simulink model "ParameterIdentification"  (R2024b)
settings: Solver=FixedStepAuto  StartTime=0.0  StopTime=3  FixedStep=1e-6  MaxStep=1e-6  RelTol=1e-3
undefined symbols (not defined in the file): F1, Period, Pn, Ts, U_ref, Udc
libraries: My_library x3, spsDCVoltageSourceLib x1, spsGroundLib x1, simulink x1, spsPermanentMagnetSynchronousMachineLib x1, spsTwoLevelConverterLib x1, sps_lib x1
(part 1 of 2)
settings Model: DataDictionary=Based_FOC_Data.sldd  Creator=sa127  LastModifiedBy=sa127
settings OptimizationCC: DefaultParameterBehavior=Inlined  UseDivisionForNetSlopeComputation=on  GainParamInheritBuiltInType=on  UseFloatMulNetSlope=on  InlineInvariantSignals=on  PassReuseOutputArgsAs=Individual arguments  ZeroExternalMemoryAtStartup=off  ZeroInternalMemoryAtStartup=off  NoFixptDivByZeroProtection=on  EfficientFloat2IntCast=on  LifeSpan=1  OptimizeBlockOrder=speed  DifferentSizesBufferReuse=on  MultiThreadedLoops=on  EfficientTunableParamExpr=on
settings DebuggingCC: ParamSuppressDoubleToSinglePrecisionLossMsg=on  ParameterTunabilityLossMsg=error
settings HardwareCC: ProdBitPerPointer=32  ProdBitPerSizeT=32  ProdBitPerPtrDiffT=32  ProdLargestAtomicInteger=Long  ProdLargestAtomicFloat=Double  ProdWordSize=32  ProdLongLongMode=on  ProdHWDeviceType=ARM Compatible->ARM Cortex-M
settings SFSimCC: MATLABDynamicMemAlloc=off
settings RTWCC: Description=Embedded Coder  SystemTargetFile=ert.tlc  TemplateMakefile=ert_default_tmf  GenerateReport=on  IncludeHyperlinkInReport=on  LaunchReport=on  GenerateTraceInfo=on  GenerateTraceReport=on  GenerateTraceReportSl=on  GenerateTraceReportSf=on  GenerateTraceReportEml=on  GenerateWebview=on  GenerateCodeMetricsReport=on  GenerateCodeReplacementReport=on
settings CodeAppCC: ForceParamTrailComments=on  IgnoreCustomStorageClasses=off  OperatorAnnotations=on  SimulinkDataObjDesc=on  SFDataObjDesc=on  CustomSymbolStrGlobalVar=rt$N$M  CustomSymbolStrType=$N$M  CustomSymbolStrFcn=$N$M$F  CustomSymbolStrMacro=$N$M  InsertBlockDesc=on
settings ERTTargetCC: TargetLangStandard=C99 (ISO)  CodeReplacementLibrary=ARM Cortex-M  GenerateSampleERTMain=on  IncludeMdlTerminateFcn=off  CombineSignalStateStructs=on  SupportComplex=off  SupportNonInlinedSFcns=on  ERTCustomFileTemplate=example_file_process.tlc  ERTFilePackagingFormat=CompactWithDataFile

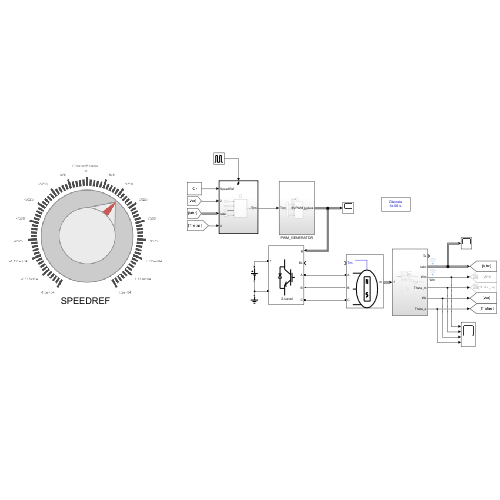
[thumbnail: Simulink's stored preview of the top-level diagram]
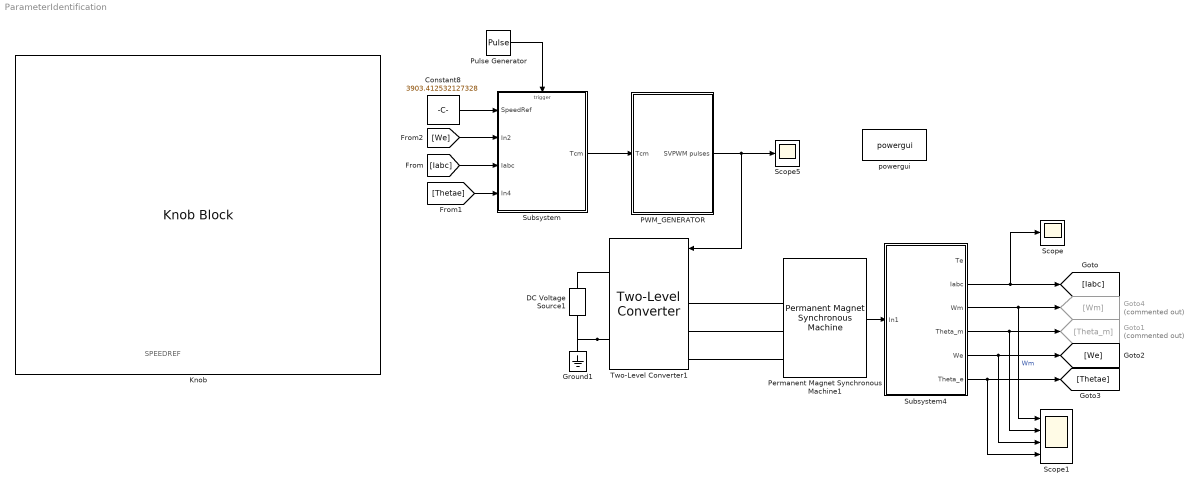
== system ParameterIdentification ==
  note: SPEEDREF
  Constant8 : Constant  Value=3903.412532127328
  DC Voltage Source1 : spsDCVoltageSourceLib/DC Voltage Source  Amplitude=300  Measurements=None
  Goto1 : Goto  Commented=on  GotoTag=Theta_m
  Goto4 : Goto  Commented=on  GotoTag=Wm
  Ground1 : spsGroundLib/Ground  LConnTagsString=a
  Knob : KnobBlock  ScaleMin=-15000  ScaleMax=15000
  PWM_GENERATOR : Subsystem
  Permanent Magnet Synchronous Machine1 : spsPermanentMagnetSynchronousMachineLib/Permanent Magnet Synchronous Machine  NbPhases=3  FluxDistribution=Sinusoidal  RotorType=Salient-pole  MechanicalLoad=Torque Tm  PresetModel="04:  6 Nm 300 Vdc 4500 RPM - 6 Nm"  ShowDetailedParameters=on  MeasurementBus=on  Resistance=0.62  Inductance=8.5e-3  dqInductances=[0.001971 0.002179]  La=0.002075  MachineConstant=Flux linkage established by magnets (V.s)  Flux=0.08627  VoltageCst=67.038  TorqueCst=0.5544  Flat=120  Mechanical=[0.0003617 9.444e-05 4 0]  PolePairs=4  InitialConditions=[0,0, 0,0]  InitialConditions5ph=[0 0 0 0 0 0]  RefAngle=Aligned with phase A axis (original Park)  IterativeDiscreteModel=Trapezoidal non iterative  TsBlock=-1  TsPowergui=0
  Pulse Generator : DiscretePulseGenerator  PulseType=Time based  Period=0.0001  PulseWidth=50
  Scope : Scope
  Scope1 : Scope  NumInputPorts=4
  Scope5 : Scope
  Subsystem : Subsystem
  Subsystem4 : Subsystem
  Two-Level Converter1 : spsTwoLevelConverterLib/Two-Level Converter  ModelType=Switching function  Ron=1e-3  Rs=1e6  Cs=inf  Vforward=[0,0]  Ron_Diode=1e-3  Rs_Diode=1e6  Cs_Diode=inf  Vf_Diode=1e-3  Rs_CurrentSource=inf  Ron_ACsource=1e-3
      settings: LibrarySourceBlock=sps_lib/Power Electronics/Two-Level Converter
  powergui : sps_lib/powergui  Priority=1  SimulationMode=Discrete  SampleTime=0.000001  frequency=60  Iterations=50  frequencyindice=0  Pbase=100e6  ErrMax=1e-4  UnitsV=kV  UnitsW=MW  buscounter=0  FunctionMessages=off  echomessages=off  EnableUseOfTLC=off  CurrentSourceSwitches=off  DisableSnubberDevices=off  DisableRonSwitches=off  DisableVfSwitches=off  DisplayEquations=off  AutomaticDiscreteSolvers=off  SolverType=Tustin/Backward Euler (TBE)  Interpol=off  ExternalGateDelay=off  methode=off  Ts=100  x0status=blocks  SPID=on  SwTol=0  HookPort=off  NonlinearTolerance=1e-4  nMaxIteration=100  ContinueOnMaxIteration=off  RestoreLinks=warning  ResistiveCurrentMeasurement=off  Frange=[0:2:500]  Ylog=off  Xlog=on  ShowGrid=off  save=off  variable=ZData  structure=0  ZoomFFT=off  StartTime=0.0  cycles=1  DisplayStyle=1  fundamental=60  FreqAxis=off  MaxFrequency=1000  frequencyindicesteady=1  RmsSteady=1  display=off
  wires:
  Permanent Magnet Synchronous Machine1/1 -> Subsystem4/1(In1)
  Subsystem4/2(Iabc) -> Scope/1, [Iabc]
  Subsystem4/3(Wm) -> Scope1/1, Goto4/1  "Wm"
  Subsystem4/4(Theta_m) -> Goto1/1, Scope1/2
  Subsystem4/5(We) -> Scope1/3, [We]
  Subsystem4/6(Theta_e) -> Scope1/4, [Thetae]
  PWM_GENERATOR/1(SVPWM pulses) -> Scope5/1, Two-Level Converter1/1
  Constant8/1 -> Subsystem/1(SpeedRef)
  [We] -> Subsystem/2(In2)
  [Iabc] -> Subsystem/3(Iabc)
  [Thetae] -> Subsystem/4(In4)
  Pulse Generator/1 -> Subsystem/Trigger
  Subsystem/1(Tcm) -> PWM_GENERATOR/1(Tcm)
  connections:
  Two-Level Converter1/RConn2 -- DC Voltage Source1/LConn1 -- Ground1/LConn1
  Two-Level Converter1/LConn2 -- Permanent Magnet Synchronous Machine1/LConn2
  Two-Level Converter1/LConn1 -- Permanent Magnet Synchronous Machine1/LConn1
  Two-Level Converter1/LConn3 -- Permanent Magnet Synchronous Machine1/LConn3
  DC Voltage Source1/RConn1 -- Two-Level Converter1/RConn1

== system ParameterIdentification/PWM_GENERATOR ==
  Tcm : Inport
  Demux : Demux  Outputs=3
  Scope1 : Scope  NumInputPorts=3
  Subsystem1 : Subsystem
  SVPWM pulses : Outport
  wires:
  Demux/1 -> Subsystem1/1(Tcm1), Scope1/1
  Demux/2 -> Subsystem1/2(Tcm2), Scope1/2
  Demux/3 -> Subsystem1/3(Tcm3), Scope1/3
  Subsystem1/1(SVPWM pulses) -> SVPWM pulses/1
  Tcm/1 -> Demux/1

== system ParameterIdentification/Subsystem ==
  SpeedRef : Inport
  In2 : Inport  Port=2
  Iabc : Inport  Port=3
  In4 : Inport  Port=4
  Trigger : TriggerPort  VariantControl=(inherit)  PortDimensions=1
  Sensorless : Subsystem
  Tcm : Outport
  wires:
  SpeedRef/1 -> Sensorless/1(SpeedRef)
  In2/1 -> Sensorless/2(In2)
  In4/1 -> Sensorless/4(In4)
  Iabc/1 -> Sensorless/3(Iabc)
  Sensorless/1(Tcm) -> Tcm/1

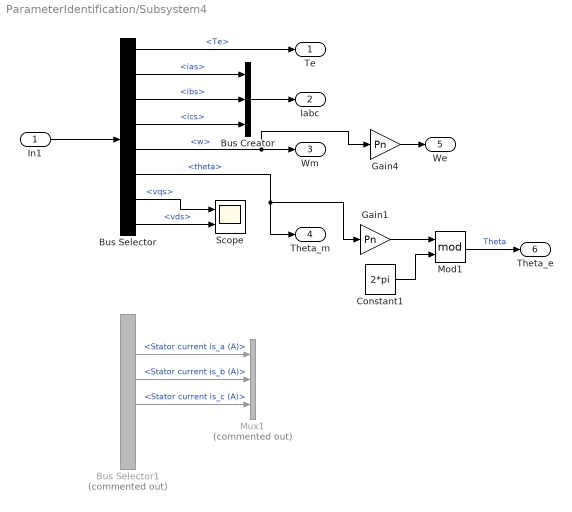
== system ParameterIdentification/Subsystem4 ==
  In1 : Inport
  Bus Creator : BusCreator  Inputs=3
  Bus Selector : BusSelector  OutputSignals=Te,ias,ibs,ics,w,theta,vqs,vds
  Bus Selector1 : BusSelector  Commented=on  OutputSignals=Electromagnetic torque Te (N*m),Stator current is_a (A),Stator current is_b (A),Stator current is_c (A),Rotor speed wm (rad/s),Rotor angle thetam (rad)
  Constant1 : Constant  Value=2*pi
  Gain1 : Gain  Gain=Pn
  Gain4 : Gain  Gain=Pn
  Mod1 : Math  Operator=mod
  Mux1 : Mux  Commented=on  Inputs=3
  Scope : Scope  NumInputPorts=2
  Te : Outport
  Iabc : Outport  Port=2
  Wm : Outport  Port=3
  Theta_m : Outport  Port=4
  We : Outport  Port=5
  Theta_e : Outport  Port=6
  wires:
  Bus Selector/2 -> Bus Creator/1  "<ias>"
  Bus Selector/4 -> Bus Creator/3  "<ics>"
  Bus Selector/3 -> Bus Creator/2  "<ibs>"
  Bus Selector1/4 -> Mux1/3  "<Stator current is_c (A)>"
  Bus Selector1/3 -> Mux1/2  "<Stator current is_b (A)>"
  Bus Selector1/2 -> Mux1/1  "<Stator current is_a (A)>"
  In1/1 -> Bus Selector/1
  Bus Selector/1 -> Te/1  "<Te>"
  Bus Selector/5 -> Gain4/1, Wm/1  "<w>"
  Bus Selector/6 -> Gain1/1, Theta_m/1  "<theta>"
  Bus Selector/8 -> Scope/2  "<vds>"
  Bus Selector/7 -> Scope/1  "<vqs>"
  Constant1/1 -> Mod1/2
  Gain1/1 -> Mod1/1
  Gain4/1 -> We/1
  Mod1/1 -> Theta_e/1  "Theta"
  Bus Creator/1 -> Iabc/1

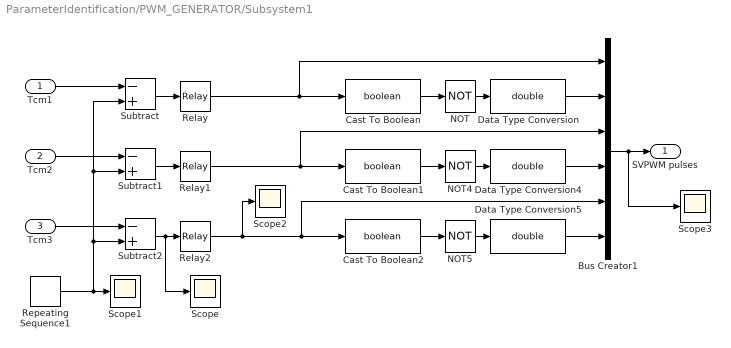
== system ParameterIdentification/PWM_GENERATOR/Subsystem1 ==
  Tcm1 : Inport
  Tcm2 : Inport  Port=2
  Tcm3 : Inport  Port=3
  Bus Creator1 : BusCreator  Inputs=6
  Cast To Boolean : DataTypeConversion  OutDataTypeStr=boolean  SaturateOnIntegerOverflow=off  RndMeth=Floor
  Cast To Boolean1 : DataTypeConversion  OutDataTypeStr=boolean  SaturateOnIntegerOverflow=off  RndMeth=Floor
  Cast To Boolean2 : DataTypeConversion  OutDataTypeStr=boolean  SaturateOnIntegerOverflow=off  RndMeth=Floor
  Data Type Conversion : DataTypeConversion  OutDataTypeStr=double  SaturateOnIntegerOverflow=off  RndMeth=Floor
  Data Type Conversion4 : DataTypeConversion  OutDataTypeStr=double  SaturateOnIntegerOverflow=off  RndMeth=Floor
  Data Type Conversion5 : DataTypeConversion  OutDataTypeStr=double  SaturateOnIntegerOverflow=off  RndMeth=Floor
  NOT : Logic  Operator=NOT  IconShape=distinctive  AllPortsSameDT=off  OutDataTypeStr=boolean
  NOT4 : Logic  Operator=NOT  IconShape=distinctive  AllPortsSameDT=off  OutDataTypeStr=boolean
  NOT5 : Logic  Operator=NOT  IconShape=distinctive  AllPortsSameDT=off  OutDataTypeStr=boolean
  Relay : Relay
  Relay1 : Relay
  Relay2 : Relay
  Repeating Sequence1 : simulink/Sources/Repeating Sequence  rep_seq_t=[0 Ts/2 Ts]  rep_seq_y=[0 Period/2 0]
  Scope{,1..3} (4 alike) : Scope
  Subtract : Sum  Inputs=-+
  Subtract1 : Sum  Inputs=-+
  Subtract2 : Sum  Inputs=-+
  SVPWM pulses : Outport
  wires:
  Tcm3/1 -> Subtract2/1
  Cast To Boolean/1 -> NOT/1
  Subtract/1 -> Relay/1
  Relay2/1 -> Scope2/1, Bus Creator1/5, Cast To Boolean2/1
  Subtract2/1 -> Scope/1, Relay2/1
  Cast To Boolean2/1 -> NOT5/1
  Subtract1/1 -> Relay1/1
  Repeating Sequence1/1 -> Subtract2/2, Subtract1/2, Subtract/2, Scope1/1
  Tcm1/1 -> Subtract/1
  NOT/1 -> Data Type Conversion/1
  Cast To Boolean1/1 -> NOT4/1
  Bus Creator1/1 -> Scope3/1, SVPWM pulses/1
  NOT5/1 -> Data Type Conversion5/1
  Relay1/1 -> Bus Creator1/3, Cast To Boolean1/1
  Relay/1 -> Bus Creator1/1, Cast To Boolean/1
  Tcm2/1 -> Subtract1/1
  Data Type Conversion5/1 -> Bus Creator1/6
  Data Type Conversion/1 -> Bus Creator1/2
  NOT4/1 -> Data Type Conversion4/1
  Data Type Conversion4/1 -> Bus Creator1/4

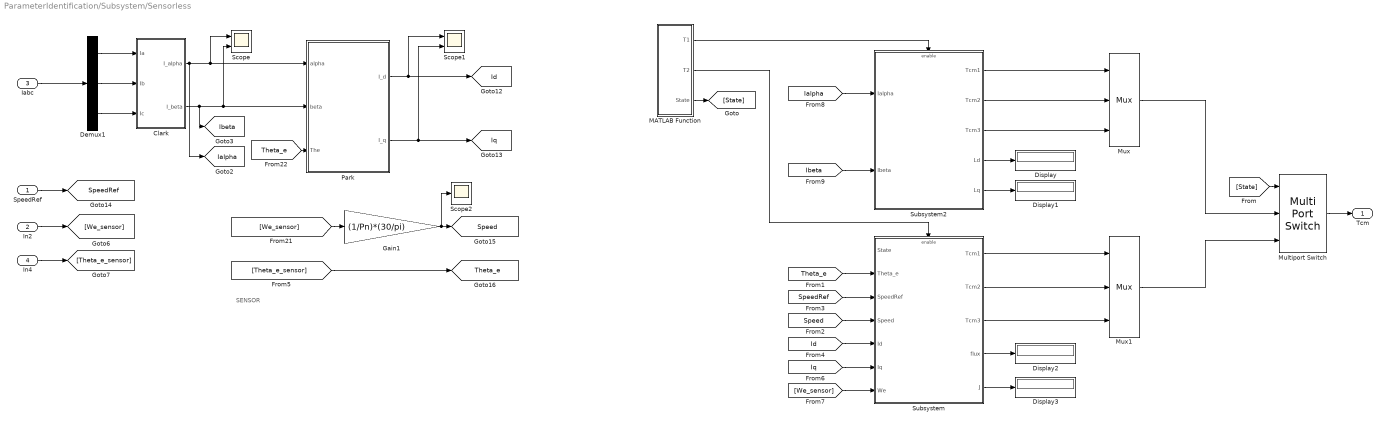
== system ParameterIdentification/Subsystem/Sensorless ==
  note: SENSOR
  SpeedRef : Inport
  In2 : Inport  Port=2
  Iabc : Inport  Port=3
  In4 : Inport  Port=4
  Clark : Subsystem
  Demux1 : Demux  Outputs=3
  Display{,1..3} (4 alike) : Display
  Gain1 : Gain  Gain=(1/Pn)*(30/pi)
  MATLAB Function : MATLAB Function  TreatAsAtomicUnit=on
  Multiport Switch : MultiPortSwitch  Inputs=2  SaturateOnIntegerOverflow=off  InputSameDT=off
  Mux : Mux  Inputs=3
  Mux1 : Mux  Inputs=3
  Park : Subsystem
  Scope : Scope  NumInputPorts=2
  Scope1 : Scope  NumInputPorts=2
  Scope2 : Scope
  Subsystem : Subsystem
  Subsystem2 : Subsystem
  Tcm : Outport
  tag scope: Ialpha=global, Ibeta=global, Id=global, Iq=global, Speed=global, SpeedRef=global, Theta_e=global
  wires:
  Park/1(I_d) -> [Id], Scope1/1
  Demux1/3 -> Clark/3(Ic)
  Demux1/1 -> Clark/1(Ia)
  Iabc/1 -> Demux1/1
  Clark/1(I_alpha) -> [Ialpha], Scope/1, Park/1(alpha)
  Clark/2(I_beta) -> [Ibeta], Scope/2, Park/2(beta)
  Park/2(I_q) -> [Iq], Scope1/2
  Demux1/2 -> Clark/2(Ib)
  [We_sensor] -> Gain1/1
  In2/1 -> [We_sensor]
  In4/1 -> [Theta_e_sensor]
  SpeedRef/1 -> [SpeedRef]
  Gain1/1 -> Scope2/1, [Speed]
  [Theta_e_sensor] -> [Theta_e]
  [Theta_e] -> Park/3(The)
  Mux/1 -> Multiport Switch/2
  Mux1/1 -> Multiport Switch/3
  Subsystem/1(Tcm1) -> Mux1/1
  Subsystem/2(Tcm2) -> Mux1/2
  Subsystem/3(Tcm3) -> Mux1/3
  MATLAB Function/2(T2) -> Subsystem/Enable
  MATLAB Function/3(State) -> [State]
  [State] -> Multiport Switch/1
  [Theta_e] -> Subsystem/2(Theta_e)
  [SpeedRef] -> Subsystem/3(SpeedRef)
  [Speed] -> Subsystem/4(Speed)
  [Id] -> Subsystem/5(Id)
  [Iq] -> Subsystem/6(Iq)
  [We_sensor] -> Subsystem/7(We)
  Multiport Switch/1 -> Tcm/1
  [Ialpha] -> Subsystem2/1(Ialpha)
  [Ibeta] -> Subsystem2/2(Ibeta)
  Subsystem2/1(Tcm1) -> Mux/1
  Subsystem2/2(Tcm2) -> Mux/2
  Subsystem2/3(Tcm3) -> Mux/3
  MATLAB Function/1(T1) -> Subsystem2/Enable
  Subsystem2/4(Ld) -> Display/1
  Subsystem2/5(Lq) -> Display1/1
  Subsystem/4(flux) -> Display2/1
  Subsystem/5(J) -> Display3/1

== system ParameterIdentification/Subsystem/Sensorless/Clark ==
  Ia : Inport
  Ib : Inport  Port=2
  Ic : Inport  Port=3
  Fcn : Fcn  Expr=(u(1)-0.5*u(2)-0.5*u(3))*2/3
  Fcn1 : Fcn  Expr=(sqrt(3)/2*u(2)-sqrt(3)/2*u(3))*2/3
  Mux : Mux  Inputs=3
  I_alpha : Outport
  I_beta : Outport  Port=2
  wires:
  Ib/1 -> Mux/2
  Fcn1/1 -> I_beta/1
  Ic/1 -> Mux/3
  Mux/1 -> Fcn1/1, Fcn/1
  Fcn/1 -> I_alpha/1
  Ia/1 -> Mux/1

== system ParameterIdentification/Subsystem/Sensorless/Park ==
  alpha : Inport
  beta : Inport  Port=2
  The : Inport  Port=3
  Fcn : Fcn  Expr=cos(u(3))*u(1)+sin(u(3))*u(2)
  Fcn1 : Fcn  Expr=-sin(u(3))*u(1)+cos(u(3))*u(2)
  Mux : Mux  Inputs=3
  I_d : Outport
  I_q : Outport  Port=2
  wires:
  Fcn/1 -> I_d/1
  Fcn1/1 -> I_q/1
  The/1 -> Mux/3
  alpha/1 -> Mux/1
  Mux/1 -> Fcn1/1, Fcn/1
  beta/1 -> Mux/2

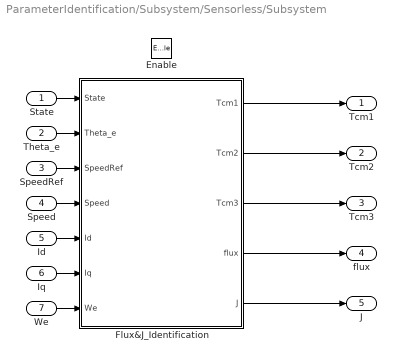
== system ParameterIdentification/Subsystem/Sensorless/Subsystem ==
  State : Inport
  Theta_e : Inport  Port=2
  SpeedRef : Inport  Port=3
  Speed : Inport  Port=4
  Id : Inport  Port=5
  Iq : Inport  Port=6
  We : Inport  Port=7
  Enable : EnablePort
  Flux&J_Identification : Subsystem
  Tcm1 : Outport
  Tcm2 : Outport  Port=2
  Tcm3 : Outport  Port=3
  flux : Outport  Port=4
  J : Outport  Port=5
  wires:
  Flux&J_Identification/1(Tcm1) -> Tcm1/1
  Flux&J_Identification/2(Tcm2) -> Tcm2/1
  State/1 -> Flux&J_Identification/1(State)
  Flux&J_Identification/3(Tcm3) -> Tcm3/1
  Theta_e/1 -> Flux&J_Identification/2(Theta_e)
  We/1 -> Flux&J_Identification/7(We)
  Iq/1 -> Flux&J_Identification/6(Iq)
  Id/1 -> Flux&J_Identification/5(Id)
  Speed/1 -> Flux&J_Identification/4(Speed)
  SpeedRef/1 -> Flux&J_Identification/3(SpeedRef)
  Flux&J_Identification/4(flux) -> flux/1
  Flux&J_Identification/5(J) -> J/1

== system ParameterIdentification/Subsystem/Sensorless/Subsystem2 ==
  Ialpha : Inport
  Ibeta : Inport  Port=2
  Enable : EnablePort
  Subsystem1 : Subsystem
  Tcm1 : Outport
  Tcm2 : Outport  Port=2
  Tcm3 : Outport  Port=3
  Ld : Outport  Port=4
  Lq : Outport  Port=5
  wires:
  Ialpha/1 -> Subsystem1/1(Ialpha)
  Ibeta/1 -> Subsystem1/2(Ibeta)
  Subsystem1/1(Tcm1) -> Tcm1/1
  Subsystem1/3(Tcm3) -> Tcm3/1
  Subsystem1/2(Tcm2) -> Tcm2/1
  Subsystem1/4(Ld) -> Ld/1
  Subsystem1/5(Lq) -> Lq/1

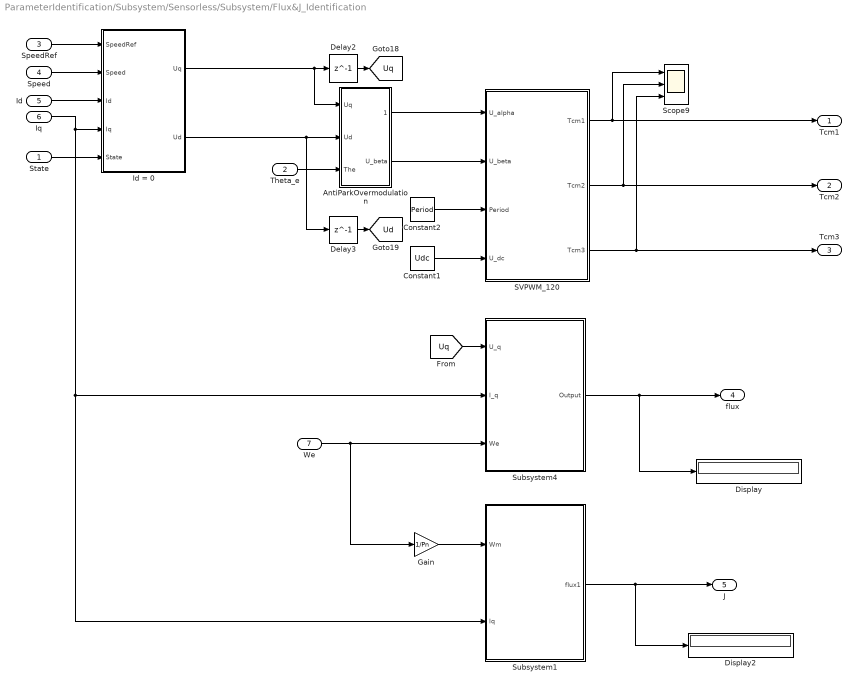
== system ParameterIdentification/Subsystem/Sensorless/Subsystem/Flux&J_Identification ==
  State : Inport
  Theta_e : Inport  Port=2
  SpeedRef : Inport  Port=3
  Speed : Inport  Port=4
  Id : Inport  Port=5
  Iq : Inport  Port=6
  We : Inport  Port=7
  AntiParkOvermodulation : Subsystem
  Constant1 : Constant  Value=Udc
  Constant2 : Constant  Value=Period
  Delay2 : Delay  DelayLength=1
  Delay3 : Delay  DelayLength=1
  Display : Display
  Display2 : Display
  Gain : Gain  Gain=1/Pn
  Id = 0 : Subsystem
  SVPWM_120 : MATLAB Function  TreatAsAtomicUnit=on
  Scope9 : Scope  NumInputPorts=3
  Subsystem1 : Subsystem
  Subsystem4 : Subsystem
  Tcm1 : Outport
  Tcm2 : Outport  Port=2
  Tcm3 : Outport  Port=3
  flux : Outport  Port=4
  J : Outport  Port=5
  tag scope: Ud=global, Uq=global
  wires:
  Iq/1 -> Subsystem4/2(I_q), Subsystem1/2(Iq), Id = 0/4(Iq)
  Id = 0/1(Uq) -> AntiParkOvermodulation/1(Uq), Delay2/1
  Speed/1 -> Id = 0/2(Speed)
  Constant2/1 -> SVPWM_120/3(Period)
  Theta_e/1 -> AntiParkOvermodulation/3(The)
  Gain/1 -> Subsystem1/1(Wm)
  Delay2/1 -> [Uq]
  SVPWM_120/3(Tcm3) -> Tcm3/1, Scope9/3
  Constant1/1 -> SVPWM_120/4(U_dc)
  [Uq] -> Subsystem4/1(U_q)
  SVPWM_120/1(Tcm1) -> Tcm1/1, Scope9/1
  Id/1 -> Id = 0/3(Id)
  SVPWM_120/2(Tcm2) -> Tcm2/1, Scope9/2
  AntiParkOvermodulation/1(U_alpha) -> SVPWM_120/1(U_alpha)
  AntiParkOvermodulation/2(U_beta) -> SVPWM_120/2(U_beta)
  Subsystem1/1(flux1) -> J/1, Display2/1
  We/1 -> Gain/1, Subsystem4/3(We)
  Subsystem4/1(Output) -> flux/1, Display/1
  Delay3/1 -> [Ud]
  Id = 0/2(Ud) -> AntiParkOvermodulation/2(Ud), Delay3/1
  SpeedRef/1 -> Id = 0/1(SpeedRef)
  State/1 -> Id = 0/5(State)

== system ParameterIdentification/Subsystem/Sensorless/Subsystem2/Subsystem1 ==
  Ialpha : Inport
  Ibeta : Inport  Port=2
  Subsystem : Subsystem
  Tcm1 : Outport
  Tcm2 : Outport  Port=2
  Tcm3 : Outport  Port=3
  Ld : Outport  Port=4
  Lq : Outport  Port=5
  wires:
  Subsystem/1(Tcm1) -> Tcm1/1
  Subsystem/3(Tcm3) -> Tcm3/1
  Subsystem/2(Tcm2) -> Tcm2/1
  Ialpha/1 -> Subsystem/1(Ialpha)
  Ibeta/1 -> Subsystem/2(Ibeta)
  Subsystem/4(Ld) -> Ld/1
  Subsystem/5(Lq) -> Lq/1

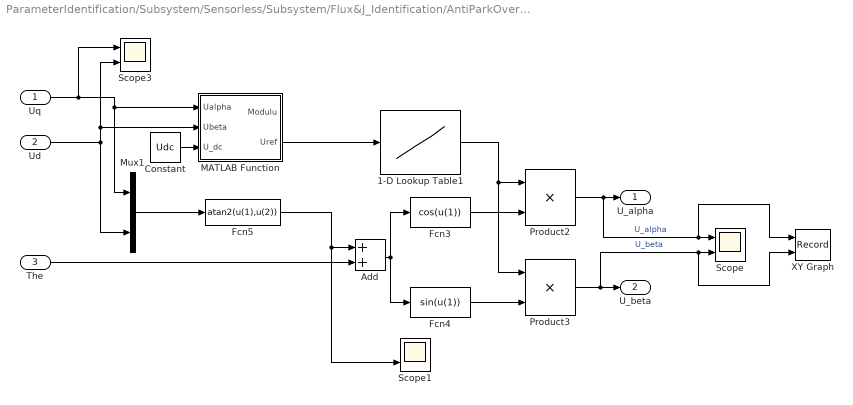
== system ParameterIdentification/Subsystem/Sensorless/Subsystem/Flux&J_Identification/AntiParkOvermodulation ==
  Uq : Inport
  Ud : Inport  Port=2
  The : Inport  Port=3
  1-D Lookup Table1 : Lookup_n-D  NumberOfTableDimensions=1  BreakpointsForDimension1=F1  Table=U_ref  ExtrapMethod=Clip  UseLastTableValue=on  InternalRulePriority=Speed  RndMeth=Simplest
  Add : Sum
  Constant : Constant  Value=Udc
  Fcn3 : Fcn  Expr=cos(u(1))
  Fcn4 : Fcn  Expr=sin(u(1))
  Fcn5 : Fcn  Expr=atan2(u(1),u(2))
  MATLAB Function : MATLAB Function  TreatAsAtomicUnit=on
  Mux1 : Mux  Inputs=2
  Product2 : Product
  Product3 : Product
  Scope : Scope  NumInputPorts=2
  Scope1 : Scope  NumInputPorts=2
  Scope3 : Scope  NumInputPorts=2
  XY Graph : Record  FileSettingsInternal="{\"entries\":[{\"content\":{\"excelSettings\":{\"content\":{},\"type\":\"Streamout.ExcelSettings\"}},\"type\":\"Streamout.FileSettingStorage\",\"uuid\":\"\"}],\"packageUris\":[\"http:\\/\\/schema.mathworks.com\\/mf0\\/streamout_blocks\\/R2020a\"],\"version\":\"1.0\"}"  Layout=[1 1]  SignalsInternal="{\"entries\":[{\"content\":{\"signals\":[{\"content\":{\"blockPath\":[],\"dimensions\":[1],\"domain\":\"\",\"lineColor\":\"#a2142f\",\"lineWidth\":2,\"port\":1,\"sid\":[\"\"],\"signalID\":1,\"signalName\":\"U_alpha\"},\"type\":\"RecordBlkView.Signal\",\"uuid\":\"\"},{\"content\":{\"blockPath\":[],\"dimensions\":[1],\"domain\":\"\",\"lineColor\":\"#139fff\",\"lineWidth\":2,\"port\":2,\"sid\":[\"\"],\"signalID\":2,\"signalName\":\"U_beta\"},\"type\":\"RecordBlkView.Signal\",\"uuid\":\"\"}]},\"type\":\"RecordBlkView.InputSignals\",\"uuid\":\"\"}],\"packageUris\":[\"http:\\/\\/schema.mathworks.com\\/mf0\\/streamout_blocks\\/R2020a\"],\"version\":\"1.0\"}"  VisualizationBindings="{\"xyplotplugin\":{\"info\":[{\"series\":[],\"subplotID\":1}]}}"  CompatibilityTag=XY
  U_alpha : Outport
  U_beta : Outport  Port=2
  wires:
  Fcn5/1 -> Scope1/2, Add/1
  Ud/1 -> MATLAB Function/2(Ubeta), Scope3/2, Mux1/2
  Fcn3/1 -> Product2/2
  Fcn4/1 -> Product3/2
  Mux1/1 -> Fcn5/1
  1-D Lookup Table1/1 -> Product2/1, Product3/1
  Product2/1 -> XY Graph/1, Scope/1, U_alpha/1  "U_alpha"
  Product3/1 -> XY Graph/2, Scope/2, U_beta/1  "U_beta"
  The/1 -> Add/2
  Add/1 -> Fcn3/1, Fcn4/1
  Constant/1 -> MATLAB Function/3(U_dc)
  Uq/1 -> Scope3/1, Mux1/1, MATLAB Function/1(Ualpha)
  MATLAB Function/2(Uref) -> 1-D Lookup Table1/1

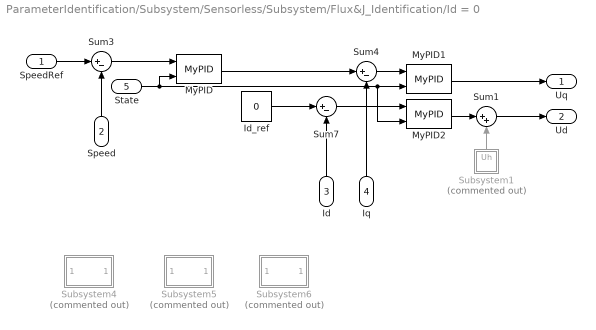
== system ParameterIdentification/Subsystem/Sensorless/Subsystem/Flux&J_Identification/Id = 0 ==
  SpeedRef : Inport
  Speed : Inport  Port=2
  Id : Inport  Port=3
  Iq : Inport  Port=4
  State : Inport  Port=5
  Id_ref : Constant  Value=0
  MyPID : My_library/MyPID  Kp=0.01  Ki=0.04  Kd=0  Ts=0.0001  max_Integral=10  min_Integral=-10  max_output=500  min_output=-500
  MyPID1 : My_library/MyPID  Kp=20  Ki=3000  Kd=0  Ts=0.0001  max_Integral=200  min_Integral=-200  max_output=200  min_output=-200
  MyPID2 : My_library/MyPID  Kp=20  Ki=3000  Kd=0  Ts=0.0001  max_Integral=200  min_Integral=-200  max_output=200  min_output=-200
  Subsystem1 : Subsystem  Commented=on
  Subsystem4 : Subsystem  Commented=on  mask{Kp=0.001, Ki=0.004, Kd=0, Ts=0.0001, max_Integral=500, min_Integral=-500, max_output=500, min_output=-500}
      mask prompts: max_Integral "积分上限"; min_Integral "积分下限"; max_output "输出上限"; min_output "输出下限"
      mask DialogControl DescTextVar Prompt: PID控制器
      mask DialogControl ParameterGroupVar Prompt: 参数
      mask Display: fprintf('MyPID');
  Subsystem5 : Subsystem  Commented=on  mask{Kp=20, Ki=3000, Kd=0, Ts=0.0001, max_Integral=500, min_Integral=-500, max_output=500, min_output=-500}
      mask prompts: max_Integral "积分上限"; min_Integral "积分下限"; max_output "输出上限"; min_output "输出下限"
      mask DialogControl DescTextVar Prompt: PID控制器
      mask DialogControl ParameterGroupVar Prompt: 参数
      mask Display: fprintf('MyPID');
  Subsystem6 : Subsystem  Commented=on  mask{Kp=20, Ki=3000, Kd=0, Ts=0.0001, max_Integral=500, min_Integral=-500, max_output=500, min_output=-500}
      mask prompts: max_Integral "积分上限"; min_Integral "积分下限"; max_output "输出上限"; min_output "输出下限"
      mask DialogControl DescTextVar Prompt: PID控制器
      mask DialogControl ParameterGroupVar Prompt: 参数
      mask Display: fprintf('MyPID');
  Sum1 : Sum  Inputs=|++
  Sum3 : Sum  Inputs=|+-
  Sum4 : Sum  Inputs=|+-
  Sum7 : Sum  Inputs=|+-
  Uq : Outport
  Ud : Outport  Port=2
  wires:
  Sum4/1 -> MyPID1/1
  Sum7/1 -> MyPID2/1
  MyPID2/1 -> Sum1/1
  Id_ref/1 -> Sum7/1
  Id/1 -> Sum7/2
  Subsystem1/1(Uh) -> Sum1/2
  Sum1/1 -> Ud/1
  SpeedRef/1 -> Sum3/1
  Sum3/1 -> MyPID/1
  Iq/1 -> Sum4/2
  Speed/1 -> Sum3/2
  MyPID/1 -> Sum4/1
  MyPID1/1 -> Uq/1
  State/1 -> MyPID2/2, MyPID1/2, MyPID/2

== system ParameterIdentification/Subsystem/Sensorless/Subsystem/Flux&J_Identification/Subsystem1 ==
  Wm : Inport
  Iq : Inport  Port=2
  Enabled Subsystem1 : Subsystem  TreatAsAtomicUnit=on
  MATLAB Function : MATLAB Function  TreatAsAtomicUnit=on
  Scope3 : Scope
  Scope4 : Scope
  Scope5 : Scope
  flux1 : Outport
  wires:
  MATLAB Function/1(T1) -> Enabled Subsystem1/Enable
  Iq/1 -> Enabled Subsystem1/2(Input1), Scope4/1
  Enabled Subsystem1/1(Output) -> flux1/1, Scope3/1
  Wm/1 -> Scope5/1, Enabled Subsystem1/1(Wm)

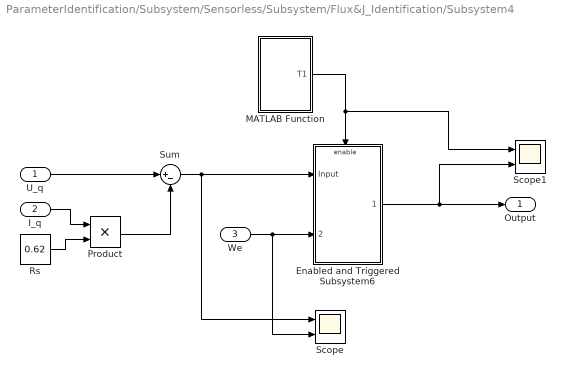
== system ParameterIdentification/Subsystem/Sensorless/Subsystem/Flux&J_Identification/Subsystem4 ==
  U_q : Inport
  I_q : Inport  Port=2
  We : Inport  Port=3
  Enabled and Triggered Subsystem6 : Subsystem  TreatAsAtomicUnit=on
  MATLAB Function : MATLAB Function  TreatAsAtomicUnit=on
  Product : Product
  Rs : Constant  Value=0.62
  Scope : Scope  NumInputPorts=2
  Scope1 : Scope  NumInputPorts=2
  Sum : Sum  Inputs=|+-
  Output : Outport
  wires:
  MATLAB Function/1(T1) -> Scope1/1, Enabled and Triggered Subsystem6/Enable
  I_q/1 -> Product/1
  Rs/1 -> Product/2
  U_q/1 -> Sum/1
  Product/1 -> Sum/2
  Sum/1 -> Scope/1, Enabled and Triggered Subsystem6/1(Input)
  We/1 -> Scope/2, Enabled and Triggered Subsystem6/2(Input1)
  Enabled and Triggered Subsystem6/1(Output) -> Scope1/2, Output/1

== system ParameterIdentification/Subsystem/Sensorless/Subsystem2/Subsystem1/Subsystem ==
  Ialpha : Inport
  Ibeta : Inport  Port=2
  Rs&Ls_Identification : Subsystem
  Tcm1 : Outport
  Tcm2 : Outport  Port=2
  Tcm3 : Outport  Port=3
  Ld : Outport  Port=4
  Lq : Outport  Port=5
  wires:
  Rs&Ls_Identification/2(Tcm2) -> Tcm2/1
  Rs&Ls_Identification/1(Tcm1) -> Tcm1/1
  Rs&Ls_Identification/3(Tcm3) -> Tcm3/1
  Ialpha/1 -> Rs&Ls_Identification/1(Ialpha)
  Ibeta/1 -> Rs&Ls_Identification/2(Ibeta)
  Rs&Ls_Identification/4(Ld) -> Ld/1
  Rs&Ls_Identification/5(Lq) -> Lq/1

== system ParameterIdentification/Subsystem/Sensorless/Subsystem/Flux&J_Identification/Id = 0/Subsystem1 ==
  MATLAB Function : MATLAB Function  TreatAsAtomicUnit=on
  Scope1 : Scope
  Uh : Outport
  tag scope: Uh=global
  wires:
  MATLAB Function/1(y) -> [Uh], Uh/1, Scope1/1

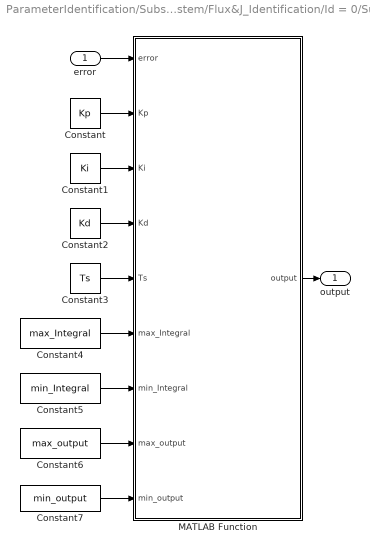
== system ParameterIdentification/Subsystem/Sensorless/Subsystem/Flux&J_Identification/Id = 0/Subsystem4 ==
  error : Inport
  Constant : Constant  Value=Kp
  Constant1 : Constant  Value=Ki
  Constant2 : Constant  Value=Kd
  Constant3 : Constant  Value=Ts
  Constant4 : Constant  Value=max_Integral
  Constant5 : Constant  Value=min_Integral
  Constant6 : Constant  Value=max_output
  Constant7 : Constant  Value=min_output
  MATLAB Function : MATLAB Function  TreatAsAtomicUnit=on
  output : Outport
  wires:
  MATLAB Function/1(output) -> output/1
  Constant2/1 -> MATLAB Function/4(Kd)
  Constant6/1 -> MATLAB Function/8(max_output)
  Constant1/1 -> MATLAB Function/3(Ki)
  error/1 -> MATLAB Function/1(error)
  Constant5/1 -> MATLAB Function/7(min_Integral)
  Constant4/1 -> MATLAB Function/6(max_Integral)
  Constant/1 -> MATLAB Function/2(Kp)
  Constant7/1 -> MATLAB Function/9(min_output)
  Constant3/1 -> MATLAB Function/5(Ts)

== system ParameterIdentification/Subsystem/Sensorless/Subsystem/Flux&J_Identification/Id = 0/Subsystem5 ==
  error : Inport
  Constant : Constant  Value=Kp
  Constant1 : Constant  Value=Ki
  Constant2 : Constant  Value=Kd
  Constant3 : Constant  Value=Ts
  Constant4 : Constant  Value=max_Integral
  Constant5 : Constant  Value=min_Integral
  Constant6 : Constant  Value=max_output
  Constant7 : Constant  Value=min_output
  MATLAB Function : MATLAB Function  TreatAsAtomicUnit=on
  output : Outport
  wires:
  MATLAB Function/1(output) -> output/1
  Constant2/1 -> MATLAB Function/4(Kd)
  Constant6/1 -> MATLAB Function/8(max_output)
  Constant1/1 -> MATLAB Function/3(Ki)
  error/1 -> MATLAB Function/1(error)
  Constant5/1 -> MATLAB Function/7(min_Integral)
  Constant4/1 -> MATLAB Function/6(max_Integral)
  Constant/1 -> MATLAB Function/2(Kp)
  Constant7/1 -> MATLAB Function/9(min_output)
  Constant3/1 -> MATLAB Function/5(Ts)

== system ParameterIdentification/Subsystem/Sensorless/Subsystem/Flux&J_Identification/Id = 0/Subsystem6 ==
  error : Inport
  Constant : Constant  Value=Kp
  Constant1 : Constant  Value=Ki
  Constant2 : Constant  Value=Kd
  Constant3 : Constant  Value=Ts
  Constant4 : Constant  Value=max_Integral
  Constant5 : Constant  Value=min_Integral
  Constant6 : Constant  Value=max_output
  Constant7 : Constant  Value=min_output
  MATLAB Function : MATLAB Function  TreatAsAtomicUnit=on
  output : Outport
  wires:
  Constant3/1 -> MATLAB Function/5(Ts)
  Constant7/1 -> MATLAB Function/9(min_output)
  Constant/1 -> MATLAB Function/2(Kp)
  Constant4/1 -> MATLAB Function/6(max_Integral)
  Constant5/1 -> MATLAB Function/7(min_Integral)
  error/1 -> MATLAB Function/1(error)
  Constant1/1 -> MATLAB Function/3(Ki)
  Constant6/1 -> MATLAB Function/8(max_output)
  Constant2/1 -> MATLAB Function/4(Kd)
  MATLAB Function/1(output) -> output/1

== system ParameterIdentification/Subsystem/Sensorless/Subsystem/Flux&J_Identification/Subsystem1/Enabled Subsystem1 ==
  Wm : Inport
  Input1 : Inport  Port=2
  Enable : EnablePort
  Display1 : Display
  Gain : Gain  Gain=9.444e-5
  Gain4 : Gain  Gain=1.5*4*0.08627
  MATLAB Function1 : MATLAB Function  TreatAsAtomicUnit=on
  Scope2 : Scope
  Sum : Sum  Inputs=-+|
  Output : Outport
  wires:
  MATLAB Function1/1(J) -> Display1/1, Output/1, Scope2/1
  Sum/1 -> MATLAB Function1/2(u2)
  Input1/1 -> Gain4/1
  Gain/1 -> Sum/1
  Gain4/1 -> Sum/2
  Wm/1 -> MATLAB Function1/1(u1), Gain/1

== system ParameterIdentification/Subsystem/Sensorless/Subsystem/Flux&J_Identification/Subsystem4/Enabled and Triggered Subsystem6 ==
  Input : Inport
  Input1 : Inport  Port=2
  Enable : EnablePort
  Display : Display
  MATLAB Function : MATLAB Function  TreatAsAtomicUnit=on
  Output : Outport
  wires:
  Input/1 -> MATLAB Function/1(u1)
  Input1/1 -> MATLAB Function/2(u2)
  MATLAB Function/1(flux) -> Output/1, Display/1

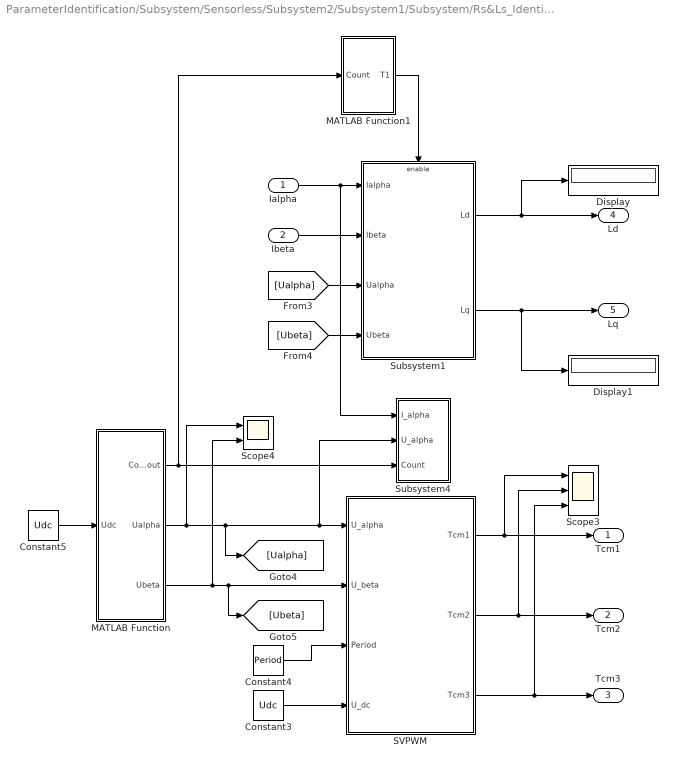
== system ParameterIdentification/Subsystem/Sensorless/Subsystem2/Subsystem1/Subsystem/Rs&Ls_Identification ==
  Ialpha : Inport
  Ibeta : Inport  Port=2
  Constant3 : Constant  Value=Udc
  Constant4 : Constant  Value=Period
  Constant5 : Constant  Value=Udc
  Display : Display
  Display1 : Display
  MATLAB Function : MATLAB Function  TreatAsAtomicUnit=on
  MATLAB Function1 : MATLAB Function  TreatAsAtomicUnit=on
  SVPWM : MATLAB Function  TreatAsAtomicUnit=on
  Scope3 : Scope  NumInputPorts=3
  Scope4 : Scope  NumInputPorts=2
  Subsystem1 : Subsystem
  Subsystem4 : Subsystem
  Tcm1 : Outport
  Tcm2 : Outport  Port=2
  Tcm3 : Outport  Port=3
  Ld : Outport  Port=4
  Lq : Outport  Port=5
  wires:
  [Ubeta] -> Subsystem1/4(Ubeta)
  MATLAB Function/2(Ualpha) -> Scope4/1, [Ualpha], Subsystem4/2(U_alpha), SVPWM/1(U_alpha)
  Subsystem1/2(Lq) -> Lq/1, Display1/1
  MATLAB Function/3(Ubeta) -> Scope4/2, [Ubeta], SVPWM/2(U_beta)
  SVPWM/2(Tcm2) -> Tcm2/1, Scope3/2
  [Ualpha] -> Subsystem1/3(Ualpha)
  Constant3/1 -> SVPWM/4(U_dc)
  Ialpha/1 -> Subsystem1/1(Ialpha), Subsystem4/1(I_alpha)
  MATLAB Function/1(Count_out) -> MATLAB Function1/1(Count), Subsystem4/3(Count)
  Subsystem1/1(Ld) -> Ld/1, Display/1
  MATLAB Function1/1(T1) -> Subsystem1/Enable
  SVPWM/3(Tcm3) -> Tcm3/1, Scope3/3
  SVPWM/1(Tcm1) -> Tcm1/1, Scope3/1
  Constant5/1 -> MATLAB Function/1(Udc)
  Constant4/1 -> SVPWM/3(Period)
  Ibeta/1 -> Subsystem1/2(Ibeta)

== system ParameterIdentification/Subsystem/Sensorless/Subsystem2/Subsystem1/Subsystem/Rs&Ls_Identification/Subsystem1 ==
  Ialpha : Inport
  Ibeta : Inport  Port=2
  Ualpha : Inport  Port=3
  Ubeta : Inport  Port=4
  Enable : EnablePort
  Subsystem : Subsystem
  Ld : Outport
  Lq : Outport  Port=2
  wires:
  Ialpha/1 -> Subsystem/1(Ialpha)
  Ibeta/1 -> Subsystem/2(Ibeta)
  Subsystem/1(Ld) -> Ld/1
  Ubeta/1 -> Subsystem/4(Ubeta)
  Subsystem/2(Lq) -> Lq/1
  Ualpha/1 -> Subsystem/3(Ualpha)

== system ParameterIdentification/Subsystem/Sensorless/Subsystem2/Subsystem1/Subsystem/Rs&Ls_Identification/Subsystem4 ==
  I_alpha : Inport
  U_alpha : Inport  Port=2
  Count : Inport  Port=3
  Enabled and Triggered Subsystem : Subsystem  TreatAsAtomicUnit=on
  Enabled and Triggered Subsystem1 : Subsystem  TreatAsAtomicUnit=on
  Enabled and Triggered Subsystem2 : Subsystem  TreatAsAtomicUnit=on
  Enabled and Triggered Subsystem3 : Subsystem  TreatAsAtomicUnit=on
  Enabled and Triggered Subsystem4 : Subsystem  TreatAsAtomicUnit=on
  Enabled and Triggered Subsystem5 : Subsystem  TreatAsAtomicUnit=on
  Subsystem1 : Subsystem
      settings: PortSchema="{\"entries\":[{\"content\":{\"sides\":[{\"content\":{},\"type\":\"ConnectorPlacement.EquallySpacedRectSide\",\"uuid\":\"cc82598c-e1f7-44bf-8906-8d1115279e7b\"},{\"content\":{\"connectorIds\":[\"Out1\",\"Out2\",\"Out3\",\"Out4\",\"Out5\",\"Out6\"],\"side\":\"RIGHT\"},\"type\":\"ConnectorPlacement.EquallySpacedRectSide\",\"uuid\":\"fdb5232a-c179-4c7b-a52e-faccd29f8392\"},{\"content\":{\"connectorIds\":[\"In1\"],\"side\":\"TOP\"},\"type\":\"ConnectorPlacement.EquallySpacedRectSide\",\"uuid\":\"b65f67fe-c4a5-4422-b216-fe9defa3c84c\"}]},\"type\":\"ConnectorPlacement.EquallySpacedConnector\",\"uuid\":\"1067b95e-88f6-44b6-ad93-56d69f36853b\"}],\"packageUris\":[\"http://schema.mathworks.com/mf0/Connector/R2020b\"],\"version\":\"1.0\"}"
  wires:
  I_alpha/1 -> Enabled and Triggered Subsystem5/1(I_alpha), Enabled and Triggered Subsystem4/1(I_alpha), Enabled and Triggered Subsystem3/1(I_alpha), Enabled and Triggered Subsystem2/1(I_alpha), Enabled and Triggered Subsystem1/1(I_alpha), Enabled and Triggered Subsystem/1(I_alpha)
  Subsystem1/1(Output) -> Enabled and Triggered Subsystem/Enable
  Subsystem1/2(Output1) -> Enabled and Triggered Subsystem1/Enable
  Subsystem1/3(Output2) -> Enabled and Triggered Subsystem2/Enable
  Subsystem1/4(Output3) -> Enabled and Triggered Subsystem3/Enable
  Subsystem1/5(Output4) -> Enabled and Triggered Subsystem4/Enable
  Subsystem1/6(Output5) -> Enabled and Triggered Subsystem5/Enable
  U_alpha/1 -> Enabled and Triggered Subsystem/2(U_alpha), Enabled and Triggered Subsystem1/2(U_alpha), Enabled and Triggered Subsystem2/2(U_alpha), Enabled and Triggered Subsystem3/2(U_alpha), Enabled and Triggered Subsystem4/2(U_alpha), Enabled and Triggered Subsystem5/2(U_alpha)
  Count/1 -> Subsystem1/1(Count)

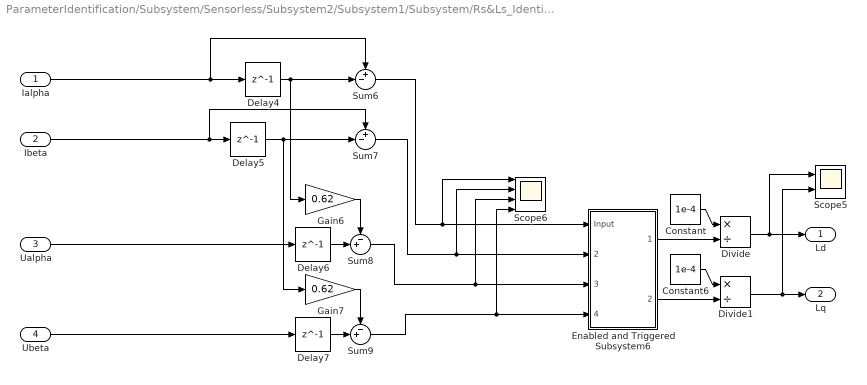
== system ParameterIdentification/Subsystem/Sensorless/Subsystem2/Subsystem1/Subsystem/Rs&Ls_Identification/Subsystem1/Subsystem ==
  Ialpha : Inport
  Ibeta : Inport  Port=2
  Ualpha : Inport  Port=3
  Ubeta : Inport  Port=4
  Constant : Constant  Value=1e-4
  Constant6 : Constant  Value=1e-4
  Delay{4..7} (4 alike) : Delay  DelayLength=1
  Divide : Product  Inputs=*/
  Divide1 : Product  Inputs=*/
  Enabled and Triggered Subsystem6 : Subsystem  TreatAsAtomicUnit=on
  Gain6 : Gain  Gain=0.62
  Gain7 : Gain  Gain=0.62
  Scope5 : Scope  NumInputPorts=2
  Scope6 : Scope  NumInputPorts=4
  Sum6 : Sum  Inputs=+-|
  Sum7 : Sum  Inputs=+-|
  Sum8 : Sum  Inputs=-+|
  Sum9 : Sum  Inputs=-+|
  Ld : Outport
  Lq : Outport  Port=2
  wires:
  Delay5/1 -> Gain7/1, Sum7/2
  Ibeta/1 -> Sum7/1, Delay5/1
  Delay4/1 -> Gain6/1, Sum6/2
  Sum9/1 -> Scope6/4, Enabled and Triggered Subsystem6/4(Input3)
  Gain6/1 -> Sum8/1
  Constant6/1 -> Divide1/1
  Sum8/1 -> Scope6/3, Enabled and Triggered Subsystem6/3(Input2)
  Ialpha/1 -> Sum6/1, Delay4/1
  Divide1/1 -> Lq/1, Scope5/2
  Sum7/1 -> Scope6/2, Enabled and Triggered Subsystem6/2(Input1)
  Delay6/1 -> Sum8/2
  Sum6/1 -> Scope6/1, Enabled and Triggered Subsystem6/1(Input)
  Divide/1 -> Ld/1, Scope5/1
  Enabled and Triggered Subsystem6/2(Output1) -> Divide1/2
  Delay7/1 -> Sum9/2
  Gain7/1 -> Sum9/1
  Constant/1 -> Divide/1
  Enabled and Triggered Subsystem6/1(Output) -> Divide/2
  Ubeta/1 -> Delay7/1
  Ualpha/1 -> Delay6/1

== system ParameterIdentification/Subsystem/Sensorless/Subsystem2/Subsystem1/Subsystem/Rs&Ls_Identification/Subsystem4/Enabled and Triggered Subsystem ==
  I_alpha : Inport
  U_alpha : Inport  Port=2
  Enable : EnablePort
  To Workspace : ToWorkspace  VariableName=I_alpha1  SampleTime=-1
      settings: Save2DSignal=2-D array (concatenate along first dimension)
  To Workspace1 : ToWorkspace  VariableName=U_alpha1  SampleTime=-1
      settings: Save2DSignal=2-D array (concatenate along first dimension)
  wires:
  I_alpha/1 -> To Workspace/1
  U_alpha/1 -> To Workspace1/1

== system ParameterIdentification/Subsystem/Sensorless/Subsystem2/Subsystem1/Subsystem/Rs&Ls_Identification/Subsystem4/Enabled and Triggered Subsystem1 ==
  I_alpha : Inport
  U_alpha : Inport  Port=2
  Enable : EnablePort
  To Workspace : ToWorkspace  VariableName=I_alpha2  SampleTime=-1
      settings: Save2DSignal=2-D array (concatenate along first dimension)
  To Workspace1 : ToWorkspace  VariableName=U_alpha2  SampleTime=-1
      settings: Save2DSignal=2-D array (concatenate along first dimension)
  wires:
  I_alpha/1 -> To Workspace/1
  U_alpha/1 -> To Workspace1/1

== system ParameterIdentification/Subsystem/Sensorless/Subsystem2/Subsystem1/Subsystem/Rs&Ls_Identification/Subsystem4/Enabled and Triggered Subsystem2 ==
  I_alpha : Inport
  U_alpha : Inport  Port=2
  Enable : EnablePort
  To Workspace : ToWorkspace  VariableName=I_alpha3  SampleTime=-1
      settings: Save2DSignal=2-D array (concatenate along first dimension)
  To Workspace1 : ToWorkspace  VariableName=U_alpha3  SampleTime=-1
      settings: Save2DSignal=2-D array (concatenate along first dimension)
  wires:
  I_alpha/1 -> To Workspace/1
  U_alpha/1 -> To Workspace1/1

== system ParameterIdentification/Subsystem/Sensorless/Subsystem2/Subsystem1/Subsystem/Rs&Ls_Identification/Subsystem4/Enabled and Triggered Subsystem3 ==
  I_alpha : Inport
  U_alpha : Inport  Port=2
  Enable : EnablePort
  To Workspace : ToWorkspace  VariableName=I_alpha4  SampleTime=-1
      settings: Save2DSignal=2-D array (concatenate along first dimension)
  To Workspace1 : ToWorkspace  VariableName=U_alpha4  SampleTime=-1
      settings: Save2DSignal=2-D array (concatenate along first dimension)
  wires:
  I_alpha/1 -> To Workspace/1
  U_alpha/1 -> To Workspace1/1

== system ParameterIdentification/Subsystem/Sensorless/Subsystem2/Subsystem1/Subsystem/Rs&Ls_Identification/Subsystem4/Enabled and Triggered Subsystem4 ==
  I_alpha : Inport
  U_alpha : Inport  Port=2
  Enable : EnablePort
  To Workspace : ToWorkspace  VariableName=I_alpha5  SampleTime=-1
      settings: Save2DSignal=2-D array (concatenate along first dimension)
  To Workspace1 : ToWorkspace  VariableName=U_alpha5  SampleTime=-1
      settings: Save2DSignal=2-D array (concatenate along first dimension)
  wires:
  I_alpha/1 -> To Workspace/1
  U_alpha/1 -> To Workspace1/1

== system ParameterIdentification/Subsystem/Sensorless/Subsystem2/Subsystem1/Subsystem/Rs&Ls_Identification/Subsystem4/Enabled and Triggered Subsystem5 ==
  I_alpha : Inport
  U_alpha : Inport  Port=2
  Enable : EnablePort
  To Workspace : ToWorkspace  VariableName=I_alpha6  SampleTime=-1
      settings: Save2DSignal=2-D array (concatenate along first dimension)
  To Workspace1 : ToWorkspace  VariableName=U_alpha6  SampleTime=-1
      settings: Save2DSignal=2-D array (concatenate along first dimension)
  wires:
  I_alpha/1 -> To Workspace/1
  U_alpha/1 -> To Workspace1/1

== system ParameterIdentification/Subsystem/Sensorless/Subsystem2/Subsystem1/Subsystem/Rs&Ls_Identification/Subsystem4/Subsystem1 ==
  Count : Inport
  MATLAB Function : MATLAB Function  TreatAsAtomicUnit=on
  Output : Outport
  Output1 : Outport  Port=2
  Output2 : Outport  Port=3
  Output3 : Outport  Port=4
  Output4 : Outport  Port=5
  Output5 : Outport  Port=6
  wires:
  MATLAB Function/1(T1) -> Output/1
  MATLAB Function/2(T2) -> Output1/1
  MATLAB Function/3(T3) -> Output2/1
  MATLAB Function/4(T4) -> Output3/1
  MATLAB Function/5(T5) -> Output4/1
  MATLAB Function/6(T6) -> Output5/1
  Count/1 -> MATLAB Function/1(Count)

== system ParameterIdentification/Subsystem/Sensorless/Subsystem2/Subsystem1/Subsystem/Rs&Ls_Identification/Subsystem1/Subsystem/Enabled and Triggered Subsystem6 ==
  Input : Inport
  Input1 : Inport  Port=2
  Input2 : Inport  Port=3
  Input3 : Inport  Port=4
  Display : Display
  Display1 : Display
  MATLAB Function : MATLAB Function  TreatAsAtomicUnit=on
  Scope1 : Scope  NumInputPorts=4
  Output : Outport
  Output1 : Outport  Port=2
  wires:
  Input/1 -> Scope1/1, MATLAB Function/1(u1)
  Input1/1 -> Scope1/2, MATLAB Function/2(u2)
  Input2/1 -> Scope1/3, MATLAB Function/3(u3)
  Input3/1 -> Scope1/4, MATLAB Function/4(u4)
  MATLAB Function/2(a2) -> Output1/1, Display1/1
  MATLAB Function/1(a1) -> Display/1, Output/1

== matlab function ParameterIdentification/Subsystem/Sensorless/Subsystem/Flux&J_Identification/AntiParkOvermodulation/MATLAB Function ==
  data: Modulu output; Ualpha input; Ubeta input; Uref output; U_dc input
function [Modulu,Uref] = fcn(Ualpha,Ubeta, U_dc)
    persistent flag;
    u = sqrt(Ualpha^2 + Ubeta^2);
    % 设定阈值
    threshold1 = U_dc * 0.6;
    threshold2 = U_dc * 2 / pi;
    % 初始化 count
    if isempty(flag)
        flag = 0;
    end

    switch(flag)
        case 0
            Uref = u;
            if(u>=threshold2)
                flag = 1;
            end

        case 1
            Uref = threshold2;
            if(u<=threshold1)
                flag = 0;
            end
        otherwise
           Uref = u; 
    end
    Modulu = u;
end

== matlab function ParameterIdentification/Subsystem/Sensorless/Subsystem/Flux&J_Identification/Id = 0/Subsystem6/MATLAB Function ==
  data: error input; output output; Kp input; Ki input; Kd input; Ts input; max_Integral input; min_Integral input; max_output input; min_output input
function output = fcn(error, Kp, Ki, Kd, Ts, max_Integral, min_Integral, max_output, min_output)
%定义参数
persistent last_error;
persistent I;

% 初始化静态变量（仅在第一次调用时执行）
if isempty(last_error)
last_error = 0;  % 假设初始误差为0
end
if isempty(I)
I = 0;           % 假设初始积分项为0
end

%比例项
P = Kp*error;

%积分项
I = I + Ki*error*Ts;
%积分限幅
if(I>=max_Integral)
    I = max_Integral;
elseif(I<=min_Integral)
    I = min_Integral;
end

%微分项
D = Kd*(error - last_error)/Ts;

%保留此次错误值
last_error = error;

%输出限幅
output = P+I+D;
if(output>=max_output)
    output = max_output;
elseif(output<=min_output)
    output = min_output;
end

== matlab function ParameterIdentification/Subsystem/Sensorless/Subsystem/Flux&J_Identification/Subsystem4/Enabled and Triggered Subsystem6/MATLAB Function ==
  data: u1 input; flux output; u2 input
function flux  = fcn(u1, u2)
u = 0.99;
persistent P;
persistent temp;

if(isempty(temp))
    temp = 1;
end
if(isempty(P))
    P = 1e5;
end

P = P/u;
P = P - (P^2)*(u2^2)/(1+u2*u2*P);
temp = temp + P*u2*(u1-u2*temp);

flux = temp;

== matlab function ParameterIdentification/Subsystem/Sensorless/Subsystem2/Subsystem1/Subsystem/Rs&Ls_Identification/SVPWM ==
  data: U_alpha input; Tcm1 output; U_beta input; Period input; U_dc input; Tcm2 output; Tcm3 output
function [Tcm1, Tcm2, Tcm3] = fcn(U_alpha, U_beta, Period, U_dc)
    % 计算 Tx, Ty
    scaleFactor = -sqrt(3) * Period / 2 / U_dc;
    Tx = scaleFactor * (sqrt(3) * 0.5 * U_alpha + 0.5 * U_beta);
    Ty = scaleFactor * U_beta;

    % 计算 Ta, Tb, Tc
    if Tx >= 0 && Ty >= 0
        Tc = 0;
        [Ta, Tb] = myfun(Tx, Ty, Period);
    elseif Tx <= Ty && Tx <= 0
        Ta = 0;
        [Tb, Tc] = myfun(Ty - Tx, -Tx, Period);
    elseif Tx > Ty && Ty <= 0
        Tb = 0;
        [Ta, Tc] = myfun(Tx - Ty, -Ty, Period);
    else
        error('Both Tx and Ty cannot be less than 0');
    end

    % 计算 T0
    T_max = max([Ta, Tb, Tc]);
    T0 = Period / 2 - T_max;

    % 计算 Tcm1, Tcm2, Tcm3
    Tcm1 = Ta + T0 / 2;
    Tcm2 = Tb + T0 / 2;
    Tcm3 = Tc + T0 / 2;

    % Tcm2 = Ta + T0 / 2;
    % Tcm3 = Tb + T0 / 2;
    % Tcm1 = Tc + T0 / 2;
end

function [T1, T2] = myfun(T3, T4, Period)
    T3_abs = abs(T3);
    T4_abs = abs(T4);
    halfPeriod = Period / 2;

    if T3_abs <= halfPeriod && T4_abs <= halfPeriod
        T1 = T3;
        T2 = T4;
    elseif T3_abs >= halfPeriod && T4_abs >= halfPeriod
        T1 = halfPeriod;
        T2 = halfPeriod;
    elseif T3_abs >= T4_abs
        if T3_abs - T4_abs >= halfPeriod
            T1 = halfPeriod;
            T2 = 0;
        else
            T1 = halfPeriod;
            T2 = halfPeriod * T4 / T3;
        end
    else
        if T4_abs - T3_abs >= halfPeriod
            T1 = 0;
            T2 = halfPeriod;
        else
            T1 = halfPeriod * T3 / T4;
            T2 = halfPeriod;
        end
    end
end

== matlab function ParameterIdentification/Subsystem/Sensorless/Subsystem/Flux&J_Identification/Subsystem4/MATLAB Function ==
  data: T1 output
function T1  = fcn()
persistent Count;
if isempty(Count)
    Count = 0;
end

if Count<1500
    Count  = Count + 1;
end

if (Count>1000)    
       T1 = 1;
else 
    T1 = 0; 
end

== matlab function ParameterIdentification/Subsystem/Sensorless/Subsystem/Flux&J_Identification/Subsystem1/Enabled Subsystem1/MATLAB Function1 ==
  settings: updateMethod=DISCRETE
  data: u1 input; J output; u2 input
function J  = fcn(u1, u2)
u = 0.99;
persistent P;
persistent temp;
persistent sum;

if(isempty(temp))
    temp = 1;
end
if(isempty(P))
    P = 1e5;
end
if(isempty(sum))
    sum = 0;
end
sum = sum + u2*0.0001;
P = P/u;
P = P - (P^2)*(sum^2)/(1+sum*sum*P);
temp = temp + P*sum*(u1-sum*temp);

J = 1/temp;

== matlab function ParameterIdentification/Subsystem/Sensorless/Subsystem2/Subsystem1/Subsystem/Rs&Ls_Identification/Subsystem4/Subsystem1/MATLAB Function ==
  data: T1 output; T2 output; T3 output; T4 output; T5 output; T6 output; Count input
function [T1,T2,T3,T4,T5,T6] = fcn(Count)
if (Count>4900&&Count<5000)    %||(u>0.39&&u<0.40)||(u>0.49&&u<0.50)||(u>0.59&&u<0.60)||(u>0.69&&u<0.70)||(u>0.79&&u<0.80)||(u>0.89&&u<0.90)
       T1 = 1;
       T2 = 0; 
       T3 = 0; 
       T4 = 0; 
       T5 = 0; 
       T6 = 0; 
elseif Count>5900&&Count<6000
       T1 = 0;
       T2 = 1; 
       T3 = 0; 
       T4 = 0; 
       T5 = 0; 
       T6 = 0;  
elseif Count>6900&&Count<7000
       T1 = 0;
       T2 = 0; 
       T3 = 1; 
       T4 = 0; 
       T5 = 0; 
       T6 = 0;  
elseif Count>7900&&Count<8000
       T1 = 0;
       T2 = 0; 
       T3 = 0; 
       T4 = 1; 
       T5 = 0; 
       T6 = 0;  
elseif Count>8900&&Count<9000
       T1 = 0;
       T2 = 0; 
       T3 = 0; 
       T4 = 0; 
       T5 = 1; 
       T6 = 0; 
elseif Count>9900&&Count<10000
       T1 = 0;
       T2 = 0; 
       T3 = 0; 
       T4 = 0; 
       T5 = 0; 
       T6 = 1; 
else 
    T1 = 0; 
    T2 = 0; 
    T3 = 0; 
    T4 = 0; 
    T5 = 0; 
    T6 = 0; 
end

== matlab function ParameterIdentification/Subsystem/Sensorless/Subsystem/Flux&J_Identification/Subsystem1/MATLAB Function ==
  data: T1 output
function T1  = fcn()
persistent Count;
if isempty(Count)
    Count = 0;
end

if Count<1000
    Count  = Count + 1;
end

if (Count<500)    
       T1 = 1;
else 
    T1 = 0; 
end

== matlab function ParameterIdentification/Subsystem/Sensorless/MATLAB Function ==
  data: T1 output; T2 output; State output
function [T1,T2,State]  = fcn()
persistent Count;
if isempty(Count)
    Count = 0;
end

if Count<30000
    Count  = Count + 1;
end

if (Count<20000) 
       State = 1;
       T1 = 1;
       T2 = 0;
elseif (Count>=20000&&Count<30000)
       State = 2;
       T2 = 1;
       T1 = 0;
else 
    State = 2;
     T1 = 0;
     T2 = 0;
end

== matlab function ParameterIdentification/Subsystem/Sensorless/Subsystem/Flux&J_Identification/Id = 0/Subsystem5/MATLAB Function ==
  data: error input; output output; Kp input; Ki input; Kd input; Ts input; max_Integral input; min_Integral input; max_output input; min_output input
function output = fcn(error, Kp, Ki, Kd, Ts, max_Integral, min_Integral, max_output, min_output)
%定义参数
persistent last_error;
persistent I;

% 初始化静态变量（仅在第一次调用时执行）
if isempty(last_error)
last_error = 0;  % 假设初始误差为0
end
if isempty(I)
I = 0;           % 假设初始积分项为0
end

%比例项
P = Kp*error;

%积分项
I = I + Ki*error*Ts;
%积分限幅
if(I>=max_Integral)
    I = max_Integral;
elseif(I<=min_Integral)
    I = min_Integral;
end

%微分项
D = Kd*(error - last_error)/Ts;

%保留此次错误值
last_error = error;

%输出限幅
output = P+I+D;
if(output>=max_output)
    output = max_output;
elseif(output<=min_output)
    output = min_output;
end

== matlab function ParameterIdentification/Subsystem/Sensorless/Subsystem2/Subsystem1/Subsystem/Rs&Ls_Identification/MATLAB Function ==
  data: Count_out output; Ualpha output; Ubeta output; Udc input
function [Count_out,Ualpha,Ubeta]= fcn(Udc)
persistent Count;
if isempty(Count)
    Count = 0;
end
Count = Count + 1;
if Count <= 2000
    Ualpha = 0;
    Ubeta = Udc/sqrt(3)*0.1;
elseif Count > 2000 && Count <= 4000
    Ualpha = Udc/sqrt(3)*0.1;
    Ubeta = 0;
elseif Count > 4000 && Count <= 5000
    Ualpha = Udc/sqrt(3)*0.1;
    Ubeta = 0;
elseif Count > 5000 && Count <= 6000
    Ualpha = Udc/sqrt(3)*0.15;
    Ubeta = 0;
elseif Count > 6000 && Count <= 7000
    Ualpha = Udc/sqrt(3)*0.20;
    Ubeta = 0;
elseif Count > 7000 && Count <= 8000
    Ualpha = Udc/sqrt(3)*0.25;
    Ubeta = 0;
elseif Count > 8000 && Count <= 9000
    Ualpha = Udc/sqrt(3)*0.30;
    Ubeta = 0;
elseif Count > 9000 && Count <= 10000
    Ualpha = Udc/sqrt(3)*0.35;
    Ubeta = 0;
elseif Count > 10000 && Count <= 12000
    Ualpha = Udc/sqrt(3)*0.1;
    Ubeta = 0;
elseif Count > 12000 && Count <= 20000
    Ud = 30;
    Uq = 0;
    theta = mod(Count,20)/20*2*pi;
    [Ualpha,Ubeta] = AntiPark(Uq,Ud,theta);
else
    Ualpha = 0;
    Ubeta = 0;
end

Count_out = Count;
end

function [Ualpha,Ubeta]= AntiPark(Uq,Ud,Theta)
Ualpha = cos(Theta)*Ud-sin(Theta)*Uq;
Ubeta = sin(Theta)*Ud+cos(Theta)*Uq;
end

== matlab function ParameterIdentification/Subsystem/Sensorless/Subsystem2/Subsystem1/Subsystem/Rs&Ls_Identification/Subsystem1/Subsystem/Enabled and Triggered Subsystem6/MATLAB Function ==
  data: u1 input; a1 output; u2 input; u3 input; u4 input; a2 output
function [a1,a2] = fcn(u1, u2, u3, u4)
u = 0.99;
persistent Ld Lq Pd Pq;
if(isempty(Ld))
    Ld = 1;
end
if(isempty(Lq))
    Lq = 1;
end
if(isempty(Pd))
    Pd = 1e5;
end
if(isempty(Pq))
    Pq = 1e5;
end
Pd = Pd/u;
Pd = Pd - (Pd^2)*(u3^2)/(1+u3*u3*Pd);
Ld = Ld + Pd*u3*(u1-u3*Ld);

Pq = Pq/u;
Pq = Pq - (Pq^2)*(u4^2)/(1+u4*u4*Pq);
Lq = Lq + Pq*u4*(u2-u4*Lq);

a1 = Ld;
a2 = Lq;

== matlab function ParameterIdentification/Subsystem/Sensorless/Subsystem2/Subsystem1/Subsystem/Rs&Ls_Identification/MATLAB Function1 ==
  data: Count input; T1 output
function T1  = fcn(Count)
if (Count>12050)    
       T1 = 1;
else
    T1 = 0; 
end

== matlab function ParameterIdentification/Subsystem/Sensorless/Subsystem/Flux&J_Identification/Id = 0/Subsystem1/MATLAB Function ==
  data: y output
function y = fcn()
persistent count;

% 初始化静态变量（仅在第一次调用时执行）
if isempty(count)
count = 1;  % 假设初始误差为0
end
%翻转电平
if(count == 1)
    count = -1;
elseif(count == -1)
    count = 1;
end

y = count*30;
